simulink model "GNC_System"  (R2025a)
settings: Solver=ode4  StartTime=0.0  StopTime=100  FixedStep=0.01  RelTol=1e-3
values from neighbouring files (symbols this model uses):
  Ixx = I_spacecraft(1,1)    [GNC_Advanced_Init.m]    (also in GNC_System_Init.m = 1200)
  Kd_x = 2 * zeta * wn * Ixx    (= 840)    [GNC_System_Init.m]
  Kp_x = Ixx * wn^2    (= 300)    [GNC_System_Init.m]
  omega0_x = 0.01    [GNC_System_Init.m]
  rw_tau = 0.02    [GNC_System_Init.m]
  tau_max = 5.0    (= 5)    [GNC_System_Init.m]
  theta0_x = 5 * pi/180    (= 0.0872664625997)    [GNC_System_Init.m]
libraries: simulink x1
settings Model: Creator=qaisokasha  LastModifiedBy=qaisokasha

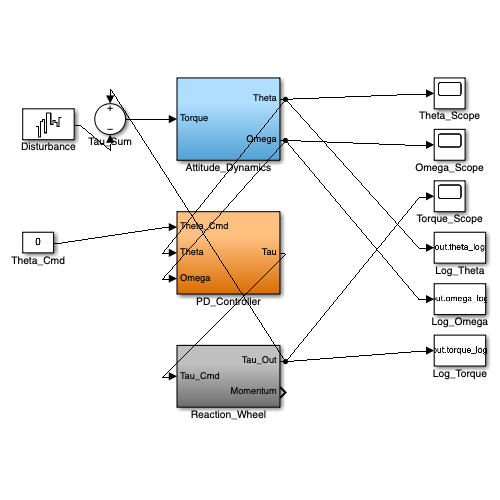
[thumbnail: Simulink's stored preview of the top-level diagram]
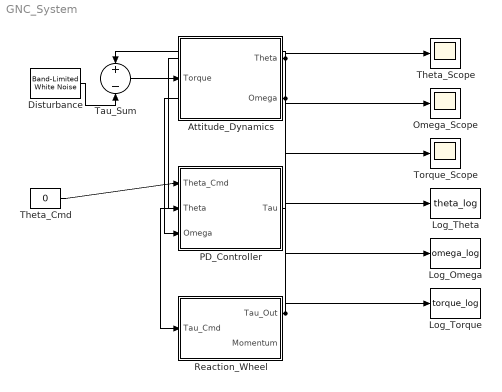
== system GNC_System ==
  Attitude_Dynamics : Subsystem
  Disturbance : simulink/Sources/Band-Limited White Noise  Cov=1e-6  Ts=0.01  seed=[23341]
  Log_Omega : ToWorkspace  VariableName=omega_log  SaveFormat=Timeseries  SampleTime=-1
  Log_Theta : ToWorkspace  VariableName=theta_log  SaveFormat=Timeseries  SampleTime=-1
  Log_Torque : ToWorkspace  VariableName=torque_log  SaveFormat=Timeseries  SampleTime=-1
  Omega_Scope : Scope
  PD_Controller : Subsystem
  Reaction_Wheel : Subsystem
  Tau_Sum : Sum  Inputs=+-
  Theta_Cmd : Constant  Value=0
  Theta_Scope : Scope
  Torque_Scope : Scope
  wires:
  Reaction_Wheel/1(Tau_Out) -> Tau_Sum/1, Torque_Scope/1, Log_Torque/1
  Disturbance/1 -> Tau_Sum/2
  Tau_Sum/1 -> Attitude_Dynamics/1(Torque)
  Attitude_Dynamics/1(Theta) -> PD_Controller/2(Theta), Theta_Scope/1, Log_Theta/1
  Attitude_Dynamics/2(Omega) -> PD_Controller/3(Omega), Omega_Scope/1, Log_Omega/1
  Theta_Cmd/1 -> PD_Controller/1(Theta_Cmd)
  PD_Controller/1(Tau) -> Reaction_Wheel/1(Tau_Cmd)

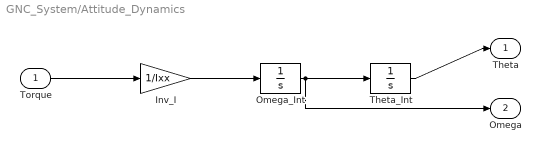
== system GNC_System/Attitude_Dynamics ==
  Torque : Inport
  Inv_I : Gain  Gain=1/Ixx
  Omega_Int : Integrator  InitialCondition=omega0_x
  Theta_Int : Integrator  InitialCondition=theta0_x
  Theta : Outport
  Omega : Outport  Port=2
  wires:
  Torque/1 -> Inv_I/1
  Inv_I/1 -> Omega_Int/1
  Omega_Int/1 -> Theta_Int/1, Omega/1
  Theta_Int/1 -> Theta/1

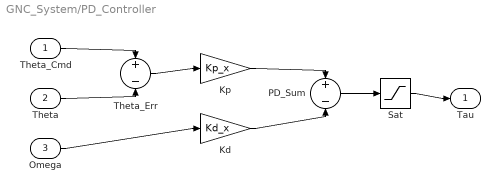
== system GNC_System/PD_Controller ==
  Theta_Cmd : Inport
  Theta : Inport  Port=2
  Omega : Inport  Port=3
  Kd : Gain  Gain=Kd_x
  Kp : Gain  Gain=Kp_x
  PD_Sum : Sum  Inputs=+-
  Sat : Saturate  UpperLimit=tau_max  LowerLimit=-tau_max
  Theta_Err : Sum  Inputs=+-
  Tau : Outport
  wires:
  Theta_Cmd/1 -> Theta_Err/1
  Theta/1 -> Theta_Err/2
  Theta_Err/1 -> Kp/1
  Omega/1 -> Kd/1
  Kp/1 -> PD_Sum/1
  Kd/1 -> PD_Sum/2
  PD_Sum/1 -> Sat/1
  Sat/1 -> Tau/1

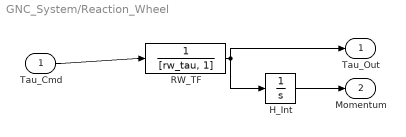
== system GNC_System/Reaction_Wheel ==
  Tau_Cmd : Inport
  H_Int : Integrator
  RW_TF : TransferFcn  Denominator=[rw_tau, 1]
  Tau_Out : Outport
  Momentum : Outport  Port=2
  wires:
  Tau_Cmd/1 -> RW_TF/1
  RW_TF/1 -> Tau_Out/1, H_Int/1
  H_Int/1 -> Momentum/1
